simulink model "Example_RPI_Xroad_task"  (Simulink 3.00)
settings: Solver=ode45  SolverMode=SingleTasking  StartTime=0.0  StopTime=10.0  RelTol=1e-3
libraries: logiclib x40, execlib x9, genlib x3, mathlib x2
settings Model: Creator=Jarda  LastModifiedBy=XPMUser

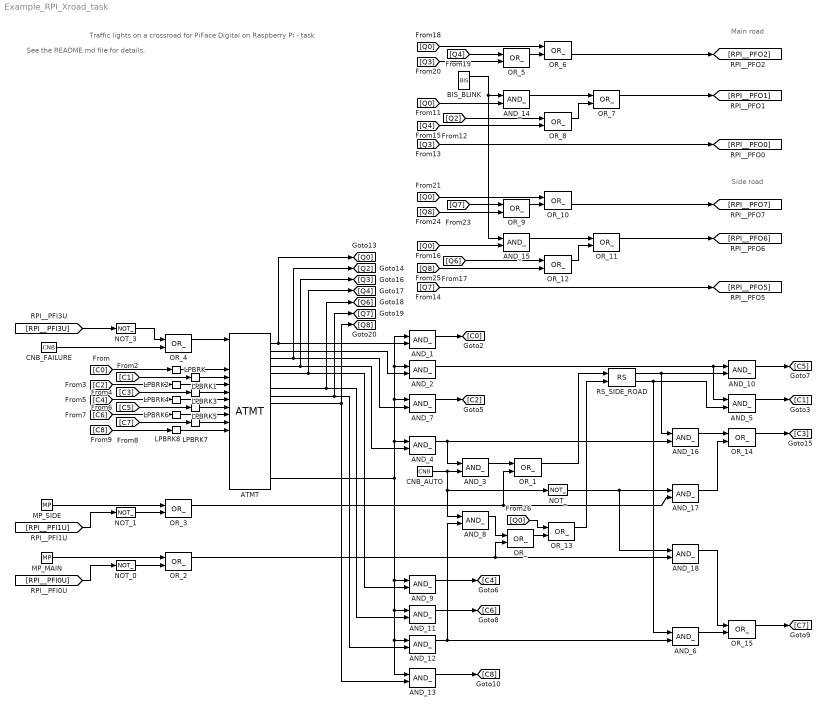
== system Example_RPI_Xroad_task ==
  note: Main road
  note: Side road
  note: Traffic lights on a crossroad for PiFace Digital on Raspberry Pi - task
  note: See the README.md file for details.
  AND_{1..18} (18 alike) : logiclib/AND_
  ATMT : logiclib/ATMT  morestps=off  ntr=9  STT=[0 0 1; 1 1 2; 2 2 3; 3 3 4; 4 4 1; 1 5 6; 6 6 7; 7 7 8;8 8 1]  touts=[1 3 2 15 2 0 2 10 2 0 0 0 0 0 0 0]
  BIS_BLINK : genlib/BIS  Y0=off  t1=1  t2=2  t3=0  t4=4  t5=5  t6=6  t7=7  t8=8  RPT=on
  CNB_AUTO : mathlib/CNB  YCN=on
  CNB_FAILURE : mathlib/CNB  YCN=off
  LPBRK{,1..8} (9 alike) : execlib/LPBRK
  MP_MAIN : genlib/MP  pwidth=1  BSTATE=off  RPTF=off
  MP_SIDE : genlib/MP  pwidth=1  BSTATE=off  RPTF=off
  NOT_{,0..1,3} (4 alike) : logiclib/NOT_
  OR_{,1..15} (16 alike) : logiclib/OR_
  RS_SIDE_ROAD : logiclib/RS
  wires:
  AND_1/1 -> [C0]
  AND_10/1 -> [C5]
  AND_11/1 -> [C6]
  AND_12/1 -> AND_6/2, AND_8/2
  AND_13/1 -> [C8]
  AND_14/1 -> OR_7/1
  AND_15/1 -> OR_11/1
  AND_16/1 -> OR_14/1
  AND_17/1 -> OR_14/2
  AND_18/1 -> OR_15/1
  AND_2/1 -> AND_10/1, AND_5/1
  AND_3/1 -> OR_1/1
  AND_4/1 -> AND_16/2, AND_3/1
  AND_5/1 -> [C1]
  AND_6/1 -> OR_15/2
  AND_7/1 -> [C2]
  AND_8/1 -> OR_/1
  AND_9/1 -> [C4]
  ATMT/1 -> AND_1/2, [Q0]
  ATMT/2 -> AND_2/2
  ATMT/3 -> AND_7/2, [Q2]
  ATMT/4 -> AND_4/2, [Q3]
  ATMT/5 -> AND_9/2, [Q4]
  ATMT/7 -> AND_11/2, [Q6]
  ATMT/8 -> AND_12/2, [Q7]
  ATMT/9 -> AND_13/2, [Q8]
  ATMT/19 -> AND_9/1, AND_11/1, AND_12/1, AND_13/1, AND_4/1, AND_7/1, AND_1/1, AND_2/1
  BIS_BLINK/1 -> AND_14/1, AND_15/1
  CNB_AUTO/1 -> AND_3/2, AND_8/1, NOT_/1
  CNB_FAILURE/1 -> OR_4/2
  [C0] -> LPBRK/1
  [Q0] -> AND_14/2
  [Q2] -> OR_8/1
  [Q3] -> [RPI__PFO0]
  [Q7] -> [RPI__PFO5]
  [Q4] -> OR_8/2
  [Q0] -> AND_15/2
  [Q6] -> OR_12/1
  [Q0] -> OR_6/1
  [Q4] -> OR_5/1
  [C1] -> LPBRK1/1
  [Q3] -> OR_5/2
  [Q0] -> OR_10/1
  [Q7] -> OR_9/1
  [Q8] -> OR_9/2
  [Q8] -> OR_12/2
  [Q0] -> OR_13/1
  [C2] -> LPBRK2/1
  [C3] -> LPBRK3/1
  [C4] -> LPBRK4/1
  [C5] -> LPBRK5/1
  [C6] -> LPBRK6/1
  [C7] -> LPBRK7/1
  [C8] -> LPBRK8/1
  LPBRK/1 -> ATMT/5
  LPBRK1/1 -> ATMT/6
  LPBRK2/1 -> ATMT/7
  LPBRK3/1 -> ATMT/8
  LPBRK4/1 -> ATMT/9
  LPBRK5/1 -> ATMT/10
  LPBRK6/1 -> ATMT/11
  LPBRK7/1 -> ATMT/12
  LPBRK8/1 -> ATMT/13
  MP_MAIN/1 -> OR_2/1
  MP_SIDE/1 -> OR_3/1
  NOT_/1 -> AND_17/1, AND_18/1
  NOT_0/1 -> OR_2/2
  NOT_1/1 -> OR_3/2
  NOT_3/1 -> OR_4/1
  OR_/1 -> OR_13/2
  OR_1/1 -> RS_SIDE_ROAD/1
  OR_10/2 -> [RPI__PFO7]
  OR_11/1 -> [RPI__PFO6]
  OR_12/1 -> OR_11/2
  OR_13/1 -> RS_SIDE_ROAD/2
  OR_14/1 -> [C3]
  OR_15/1 -> [C7]
  OR_2/1 -> AND_18/2, OR_/2
  OR_3/1 -> AND_17/2, OR_1/2
  OR_4/1 -> ATMT/1
  OR_5/1 -> OR_6/2
  OR_6/2 -> [RPI__PFO2]
  OR_7/1 -> [RPI__PFO1]
  OR_8/1 -> OR_7/2
  OR_9/1 -> OR_10/2
  [RPI__PFI0U] -> NOT_0/1
  [RPI__PFI1U] -> NOT_1/1
  [RPI__PFI3U] -> NOT_3/1
  RS_SIDE_ROAD/1 -> AND_10/2, AND_16/1
  RS_SIDE_ROAD/2 -> AND_5/2, AND_6/1
